simulink model "Sym_opt"  (R2024b)
settings: Solver=ode1  StartTime=0.0  StopTime=60  FixedStep=0.1  RelTol=1e-3
undefined symbols (not defined in the file or in its folder): Kp, rozdzielacz, Td, Ti
settings Model: Creator=bruzd  LastModifiedBy=bruzd

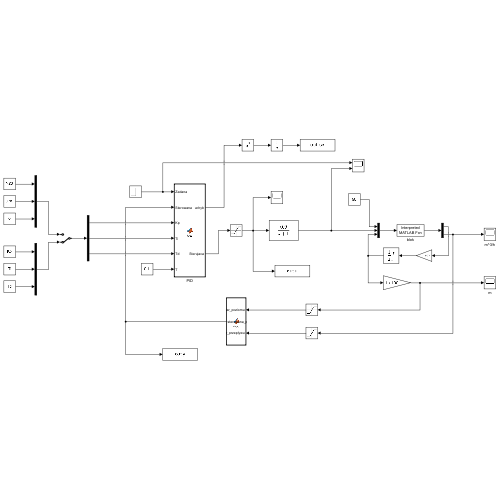
[thumbnail: Simulink's stored preview of the top-level diagram]
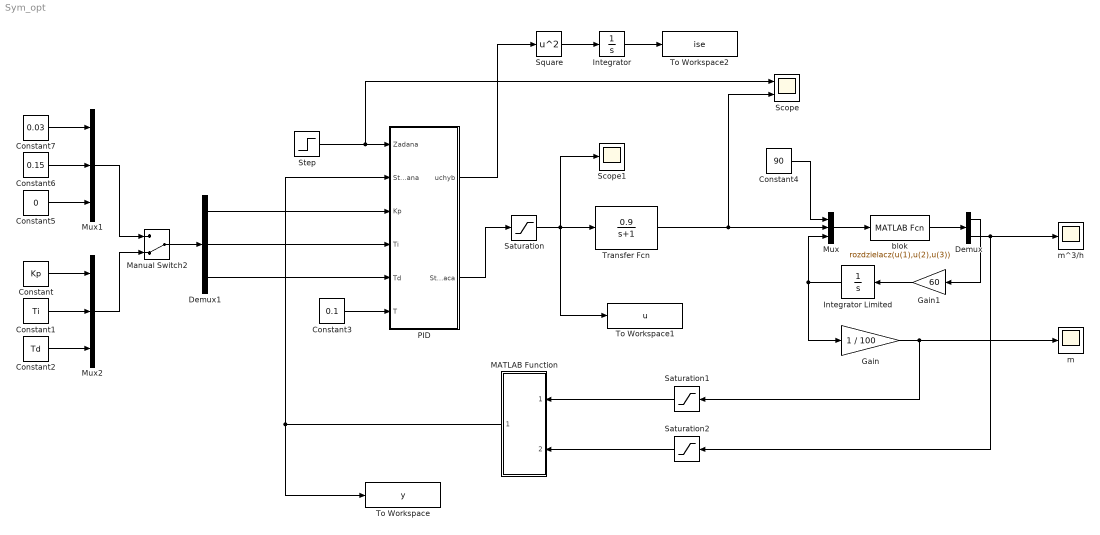
== system Sym_opt ==
  Constant : Constant  Value=Kp
  Constant1 : Constant  Value=Ti
  Constant2 : Constant  Value=Td
  Constant3 : Constant  Value=0.1
  Constant4 : Constant  Value=90
  Constant5 : Constant  Value=0
  Constant6 : Constant  Value=0.15
  Constant7 : Constant  Value=0.03
  Demux : Demux  Outputs=2
  Demux1 : Demux  Outputs=3
  Gain : Gain  Gain=1 / 100
  Gain1 : Gain  Gain=60
  Integrator : Integrator
  Integrator Limited : Integrator  InitialCondition=150  LimitOutput=on  UpperSaturationLimit=500  LowerSaturationLimit=0
  MATLAB Function : MATLAB Function  TreatAsAtomicUnit=on
  Manual Switch2 : ManualSwitch  CurrentSetting=0
  Mux : Mux  Inputs=3
  Mux1 : Mux  Inputs=3
  Mux2 : Mux  Inputs=3
  PID : MATLAB Function  TreatAsAtomicUnit=on
  Saturation : Saturate  UpperLimit=120  LowerLimit=0
  Saturation1 : Saturate  UpperLimit=5  LowerLimit=0
  Saturation2 : Saturate  UpperLimit=200  LowerLimit=0
  Scope : Scope  NumInputPorts=2
  Scope1 : Scope
  Square : Math  Operator=square
  Step : Step  Time=0  After=100  SampleTime=0
  To Workspace : ToWorkspace  VariableName=y  SaveFormat=Timeseries  SampleTime=-1
  To Workspace1 : ToWorkspace  VariableName=u  SaveFormat=Timeseries  SampleTime=-1
  To Workspace2 : ToWorkspace  VariableName=ise  SaveFormat=Timeseries  SampleTime=-1
  Transfer Fcn : TransferFcn  Numerator=[0.9]  Denominator=[1 1]
  blok : MATLABFcn  MATLABFcn=rozdzielacz(u(1),u(2),u(3))  OutputDimensions=2
  m : Scope
  m^3/h : Scope
  wires:
  Step/1 -> PID/1(Zadana), Scope/1
  Constant3/1 -> PID/6(T)
  Demux/1 -> Gain1/1
  Mux/1 -> blok/1
  blok/1 -> Demux/1
  MATLAB Function/1(sterowana_pompa) -> PID/2(Sterowana), To Workspace/1
  Constant4/1 -> Mux/1
  Gain/1 -> Saturation1/1, m/1
  Demux/2 -> Saturation2/1, m^3/h/1
  PID/2(Sterujaca) -> Saturation/1
  Transfer Fcn/1 -> Scope/2, Mux/2
  Integrator Limited/1 -> Mux/3, Gain/1
  Gain1/1 -> Integrator Limited/1
  Saturation/1 -> To Workspace1/1, Scope1/1, Transfer Fcn/1
  Saturation1/1 -> MATLAB Function/1(pomiar_poziomu)
  Saturation2/1 -> MATLAB Function/2(pomiar_przeplywu)
  PID/1(uchyb) -> Square/1
  Square/1 -> Integrator/1
  Integrator/1 -> To Workspace2/1
  Demux1/1 -> PID/3(Kp)
  Demux1/2 -> PID/4(Ti)
  Demux1/3 -> PID/5(Td)
  Constant5/1 -> Mux1/3
  Constant7/1 -> Mux1/1
  Constant6/1 -> Mux1/2
  Manual Switch2/1 -> Demux1/1
  Constant/1 -> Mux2/1
  Constant1/1 -> Mux2/2
  Constant2/1 -> Mux2/3
  Mux2/1 -> Manual Switch2/2
  Mux1/1 -> Manual Switch2/1

== matlab function Sym_opt/MATLAB Function ==
  settings: updateMethod=DISCRETE
  data: pomiar_poziomu input; pomiar_przeplywu input; sterowana_pompa output
function sterowana_pompa = fcn(pomiar_poziomu, pomiar_przeplywu)
    persistent h_poprzednie
    
    if isempty(h_poprzednie)
        h_poprzednie = 1.5;
    end

    sterowana_pompa = pomiar_przeplywu + (pomiar_poziomu - h_poprzednie) * 600 * 100;
    h_poprzednie = pomiar_poziomu;

== matlab function Sym_opt/PID ==
  settings: updateMethod=DISCRETE
  data: uchyb output; Zadana input; Sterujaca output; Sterowana input; Kp input; Ti input; Td input; T input
function [uchyb, Sterujaca] = fcn(Zadana, Sterowana, Kp, Ti, Td, T)
    persistent uchyb_poprzedni integrator

    if isempty(integrator)
        integrator = 0;
    end
    if isempty(uchyb_poprzedni)
        uchyb_poprzedni = 0;
    end

    uchyb = Zadana - Sterowana;
    integrator = integrator + uchyb * T;
    rozniczka = (uchyb - uchyb_poprzedni) / T;

    uchyb_poprzedni = uchyb;

    Sterujaca = Kp * (uchyb + (1 / Ti) * integrator + Td * rozniczka);
